simulink model "actuator"  (R2024b)
settings: Solver=VariableStepAuto  StartTime=0.0  StopTime=2  MaxStep=1e-4  RelTol=1e-3
undefined symbols (not defined in the file): act_anglelimit, act_backlash, act_ratelimit
libraries: aerolibactuator x1
settings Model: Creator=finnb  LastModifiedBy=finnb

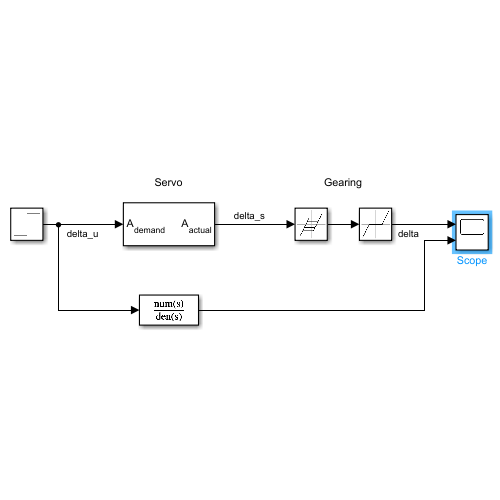
[thumbnail: Simulink's stored preview of the top-level diagram]
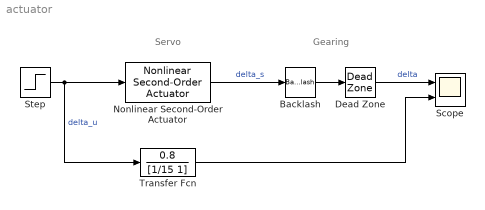
== system actuator ==
  note: Servo
  note: Gearing
  Backlash : Backlash  BacklashWidth=deg2rad(act_backlash)
  Dead Zone : DeadZone  LowerValue=-deg2rad(act_backlash)  UpperValue=deg2rad(act_backlash)
  Nonlinear Second-Order Actuator : aerolibactuator/Nonlinear Second-Order Actuator  wn_fin=act_freq  z_fin=act_damping  fin_max=deg2rad(act_anglelimit)  fin_min=-deg2rad(act_anglelimit)  fin_maxrate=deg2rad(act_ratelimit)*10  fin_act_0=0  fin_act_vel=0
  Scope : Scope  NumInputPorts=2
  Step : Step  After=0.1  SampleTime=0
  Transfer Fcn : TransferFcn  Numerator=[0.8]  Denominator=[1/15 1]
  wires:
  Step/1 -> Transfer Fcn/1, Nonlinear Second-Order Actuator/1  "delta_u"
  Backlash/1 -> Dead Zone/1
  Nonlinear Second-Order Actuator/1 -> Backlash/1  "delta_s"
  Dead Zone/1 -> Scope/1  "delta"
  Transfer Fcn/1 -> Scope/2
